simulink model "pcopy_offline_saturation"  (R2017a)
settings: Solver=FixedStepAuto  StartTime=0.0  StopTime=30  FixedStep=0.0001  RelTol=1e-3  EnableMultiTasking=on
settings Model: ExtModeTrigDuration=5000  Creator=MLevis  LastModifiedBy=Administrator
settings SolverCC: PositivePriorityOrder=on
settings DataIOCC: LimitDataPoints=on  SaveFormat=Array
settings OptimizationCC: LifeSpan=inf
settings DebuggingCC: SolverPrmCheckMsg=warning  SFUnexpectedBacktrackingDiag=warning  SFNoUnconditionalDefaultTransitionDiag=warning  SFExecutionAtInitializationDiag=none
settings HardwareCC: ProdBitPerPointer=32  ProdBitPerSizeT=32  ProdBitPerPtrDiffT=32  ProdLargestAtomicFloat=None  ProdIntDivRoundTo=Undefined  ProdEndianess=Unspecified  ProdWordSize=32  ProdHWDeviceType=32-bit Generic
settings ModelReferenceCC: PropagateSignalLabelsOutOfModel=off
settings RTWCC: SystemTargetFile=quarc_win64.tlc  TemplateMakefile=quarc_default_tmf  Description=QUARC Win64 Target
settings STFCustomTargetCC: TargetPreCompLibLocation=C:\PROGRA~3\QUARC\lib\2014a\win64\release  ConcurrentExecutionCompliant=on  GeneratePreprocessorConditionals=Disable all  SystemTargetFile=quarc_win64.tlc
settings GRTTargetCC: TargetPreCompLibLocation=C:\PROGRA~3\QUARC\lib\2014a\win64\release  TargetLangStandard=C89/C90 (ANSI)  ParMdlRefBuildCompliant=off  CompOptLevelCompliant=off  GeneratePreprocessorConditionals=Disable all  CombineOutputUpdateFcns=off  MatFileLogging=off  CPPClassGenCompliant=off  GRTInterface=on  UseToolchainInfoCompliant=off  ExtMode=on  ExtModeMexFile=quarc_comm
settings ConfigComp: CovMetricSettings=dw  CovHtmlReporting=on  CovSaveCumulativeToWorkspaceVar=on  CovSaveSingleToWorkspaceVar=on  CovExternalEMLEnable=off  CovSFcnEnable=off

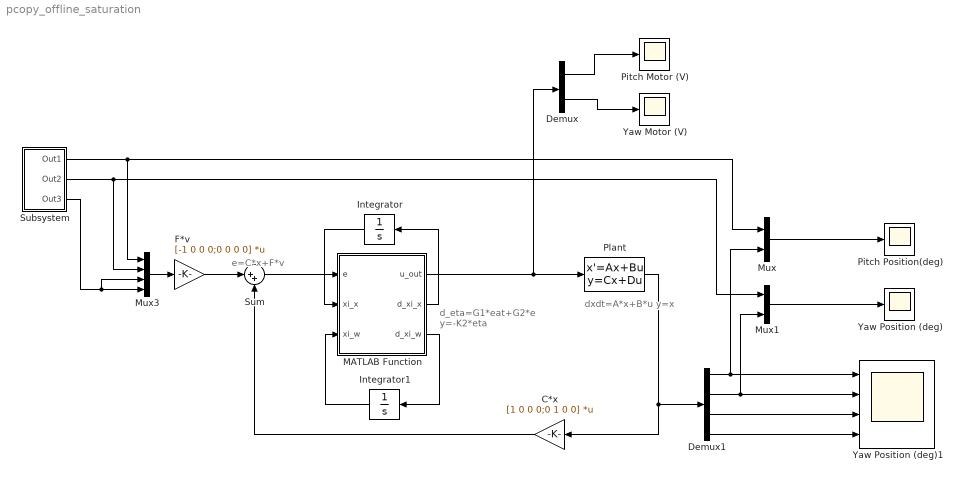
== system pcopy_offline_saturation ==
  note: dxdt=A*x+B*u
      |      y=x
  note: e=C*x+F*v
  note: d_eta=G1*eat+G2*e
      |        y=-K2*eta
  C*x : Gain  Gain=[1 0 0 0;0 1 0 0]  Multiplication=Matrix(K*u)
  Demux : Demux  Outputs=2
  Demux1 : Demux
  F*v : Gain  Gain=[-1 0 0 0;0 0 0 0]  Multiplication=Matrix(K*u)
  Integrator : Integrator  InitialCondition=[0; 1; 0; 0]
  Integrator1 : Integrator  InitialCondition=[1; 0; 0]
  MATLAB Function : MATLAB Function  TreatAsAtomicUnit=on
  Mux : Mux  Inputs=2
  Mux1 : Mux  Inputs=2
  Mux3 : Mux
  Pitch Motor (V) : Scope
  Pitch Position(deg) : Scope
  Plant : StateSpace  A=[0 0 1 0;0 0 0 1;-1.7117 0 -0.3249 0;0 0 0 -1.0004]  B=[0 0;0 0;0.0503 0.0959;-0.1228 0.1]  C=[1 0 0 0;0 1 0 0;0 0 1 0;0 0 0 1]  D=[0 0;0 0;0 0;0 0]  X0=[2;1;0;0]
  Subsystem : Subsystem
  Sum : Sum  Inputs=|++
  Yaw Motor (V) : Scope
  Yaw Position (deg) : Scope
  Yaw Position (deg)1 : Scope  NumInputPorts=4
  wires:
  Mux/1 -> Pitch Position(deg)/1
  Demux/1 -> Pitch Motor (V)/1
  Demux/2 -> Yaw Motor (V)/1
  Sum/1 -> MATLAB Function/1(e)
  Mux1/1 -> Yaw Position (deg)/1
  Mux3/1 -> F*v/1
  Subsystem/1(Out1) -> Mux3/1, Mux/1
  Subsystem/2(Out2) -> Mux3/2, Mux1/1
  Subsystem/3(Out3) -> Mux3/3, Mux3/4
  F*v/1 -> Sum/1
  C*x/1 -> Sum/2
  Plant/1 -> C*x/1, Demux1/1
  Demux1/2 -> Yaw Position (deg)1/2, Mux1/2
  Demux1/1 -> Yaw Position (deg)1/1, Mux/2
  Demux1/3 -> Yaw Position (deg)1/3
  Demux1/4 -> Yaw Position (deg)1/4
  MATLAB Function/2(d_xi_x) -> Integrator/1
  Integrator/1 -> MATLAB Function/2(xi_x)
  MATLAB Function/3(d_xi_w) -> Integrator1/1
  Integrator1/1 -> MATLAB Function/3(xi_w)
  MATLAB Function/1(u_out) -> Plant/1, Demux/1

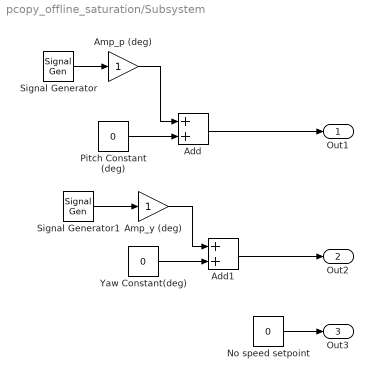
== system pcopy_offline_saturation/Subsystem ==
  Add : Sum
  Add1 : Sum
  Amp_p (deg) : Gain
  Amp_y (deg) : Gain
  No speed setpoint : Constant  Value=0
  Pitch Constant (deg) : Constant  Value=0
  Signal Generator : SignalGenerator  WaveForm=square
  Signal Generator1 : SignalGenerator  WaveForm=square
  Yaw Constant(deg) : Constant  Value=0
  Out1 : Outport
  Out2 : Outport  Port=2
  Out3 : Outport  Port=3
  wires:
  Pitch Constant (deg)/1 -> Add/2
  Signal Generator/1 -> Amp_p (deg)/1
  Add1/1 -> Out2/1
  Add/1 -> Out1/1
  Signal Generator1/1 -> Amp_y (deg)/1
  Amp_y (deg)/1 -> Add1/1
  Yaw Constant(deg)/1 -> Add1/2
  Amp_p (deg)/1 -> Add/1
  No speed setpoint/1 -> Out3/1

== matlab function pcopy_offline_saturation/MATLAB Function ==
  data: e input; u_out output; xi_x input; xi_w input; d_xi_x output; d_xi_w output
function [u_out,d_xi_x,d_xi_w] = fcn(e,xi_x,xi_w)


A=[0 0 1 0;
    0 0 0 1;
    -1.7117 0 -0.3249 0;
    0 0 0 -1.0004];
B=[0 0;
    0 0;
    0.0503 0.0959;
    -0.1228 0.1];
C=[1 0 0 0;0 1 0 0];

a1=-1.7117; a2=-0.3249; a3=-1.0004;
b1=0.0503; b2=0.0959; b3=-0.1228; b4=0.1;

c1=(a1+1)/(b1*b4/b3-b2);    % 5.2002
c2=a2/(b1*b4/b3-b2);        % 2.3739
d1=-b4/b3*c1;   % 4.2347
d2=-b4/b3*c2;   % 1.9332

% find the relationship of Xss with v, then get my_pi
my_pi = [1 0 0;0 0 0;0 1 0;0 0 0];
%my_tau = [d1 d2 0;c1 c2 0];
my_tau = [4.2347 1.9332 0;5.2002 2.3739 0];

% exosystem : v1=sin(t), v2=cos(t), v3=v3(0)
S=[0 1 0;-1 0 0;0 0 0];

% disterbance and reference signal
P=[0 0 1;0 0 2;0 0 0;1 1 1];
Q=[-1 0 0;0 0 0];

%for the saturation control
% A_tue = [A P;zeros(3,4) S];   % 7x7
% C_tue = [C Q];  % 2x7
% P0 = [-1+2i -1-2i -2+1i -2-1i -3+4i -3-4i -5];
% G = place(A_tue', C_tue', P0);
% G = G'; % 7x2
G = [-16.2034 -3.5262;1.2251 8.2511;-3.6152 45.4697;-21.7435 ...
    16.7565;-23.6270 -1.5953;-5.5222 67.1010;12.5873 10.1602];
G_1 = G(1:4,:);
G_2 = G(5:7,:);

u_out = zeros(2,1);
% controler
u_out(1:2) = sat(my_tau*xi_w + mu(xi_x - my_pi*xi_w));


d_xi_x = zeros(4, 1);
d_xi_w = zeros(3, 1);

d_xi_x(1:4) = A*xi_x + B*u_out + P*xi_w - G_1*(C*xi_x + Q*xi_w - e);

d_xi_x(1:3) = S*xi_w - G_2*(C*xi_x + Q*xi_w - e);

end


%% define the saturation function
function sat_output = sat(sat_input)
% define the maxmum allowed value of output
M = 50;
temp_output = zeros(2,1);

for icount=1:1:2
    if sat_input(icount)>M
        temp_output(icount) = M;
    elseif sat_input(icount)<-M
        temp_output(icount) = -M;
    else
        temp_output(icount) = sat_input(icount);
    end
end
sat_output = temp_output;
end


%% define the function mu:mu(0)=0
function mu_output = mu(mu_input)
% calculate the feedback gian
% A=[0 0 1 0;
%     0 0 0 1;
%     -1.7117 0 -0.3249 0;
%     0 0 0 -1.0004];
% B=[0 0;
%     0 0;
%     0.0503 0.0959;
%     -0.1228 0.1];
% P=[-7-2i -7+2i  -8+5i -8-5i];
% K=place(A,B,P);

K = [483.8793 -258.4483 104.0509 -61.7272;
     415.3003 344.2850 98.4364 64.2079];

% define rou in [0,M]
temp = zeros(4,1);
rou = 6;
for i=1:1:4
    temp(i) = (rou/2) * (1-exp(-mu_input(i)))/(1+exp(-mu_input(i)));
end
mu_output = -K*temp;
end
